simulink model "Simulacoes_lineares_naolineares"  (R2023b)
settings: Solver=ode14x  StartTime=0.0  StopTime=100  FixedStep=0.001  MaxStep=0.001  RelTol=1e-3  AbsTol=1e-3
values from neighbouring files (symbols this model uses):
  c = 0.002644555192158    (= 0.00264455519216)    [Funcoes_transferencia.m]
  carro = [K/((s+a)*(s+b))]/1000    [Funcoes_transferencia.m]
  Controlo_angulo = (46.092*(s+0.3686)*(s+5.276))/s    [Funcoes_transferencia.m]
  g = 9.8    [Funcoes_transferencia.m]
  J = 0.0001    [Funcoes_transferencia.m]
  Kd = -26.257    [Funcoes_transferencia.m]
  Kp = -26.257*6    (= -157.542)    [Funcoes_transferencia.m]
  l = 0.38    [Funcoes_transferencia.m]
  m = 0.099    [Funcoes_transferencia.m]
  s = tf('s')    [Funcoes_transferencia.m]
libraries: slpidlib x4, cstblocks x3, simulink_extras x2
settings Model: Creator=henri  LastModifiedBy=alexa
settings SolverCC: AutoScaleAbsTol=off  AlgebraicLoopSolver=TrustRegion  MaxZcPerStep=1
settings DebuggingCC: UnconnectedInputMsg=warning  UnconnectedOutputMsg=warning  UnconnectedLineMsg=warning  SymbolicDimsDataTypeCodeGenerationDiagnostic=none
settings ModelReferenceCC: EnableRefExpFcnMdlSchedulingChecks=on
settings SFSimCC: CustomCodeUndefinedFunction=UseInterfaceOnly
settings RTWCC: DLArmComputeVersion=19.05
settings SimscapeCC: SimscapeLogType=all  SimscapeLogSimulationStatistics=on  SimscapeLogDataHistory=10000

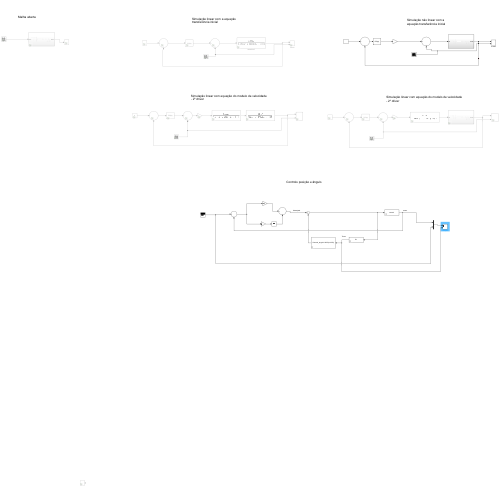
[thumbnail: Simulink's stored preview of the top-level diagram]
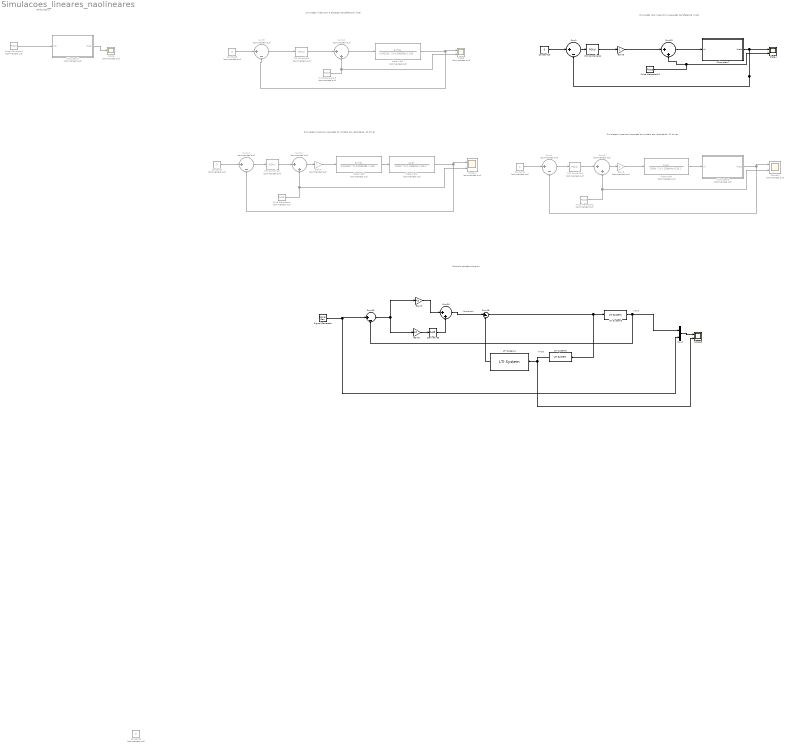
== system Simulacoes_lineares_naolineares ==
  note: Simulação linear com a equação transferência inicial
  note: Malha aberta
  note: Simulação linear com equação do modelo de velocidade - 2º driver
  note: Xdesejado
  note: Theta
  note: xcarro
  note: Controlo posição e ângulo
  note: Simulação não linear com a equação transferência inicial
  note: Simulação linear com equação do modelo de velocidade - 2º driver
  Constant{1,5..6,9} (4 alike) : Constant  Commented=on  Value=0
  Constant10 : Constant  Value=0
  Derivative3 : Derivative
  Gain4 : Gain  Commented=on
  Gain5 : Gain  Gain=Kp
  Gain6 : Gain  Gain=Kd
  Gain8 : Gain
  Gain9 : Gain  Commented=on
  LTI System3 : cstblocks/LTI System  sys=G1  IC=[]  PadeOrder=0
  LTI System4 : cstblocks/LTI System  sys=Controlo_angulo*1000/(s+1000)  IC=[]  PadeOrder=0
  LTI System5 : cstblocks/LTI System  sys=carro/s  IC=[]  PadeOrder=0
  Mux2 : Mux  Inputs=2
  PID Controller1 : slpidlib/PID Controller  Commented=on  Controller=PID  Form=Parallel  TimeDomain=Continuous-time  UseExternalTs=off  SampleTime=-1  IntegratorMethod=Forward Euler  FilterMethod=Forward Euler  ControllerParametersSource=internal  P=260.2  I=89.64  UseKiTs=off  D=46.09  N=1000  UseFilter=on  TunerSelectOption=Frequency Response Based  InitialConditionSource=internal  InitialConditionForIntegrator=0  InitialConditionForFilter=0  DifferentiatorICPrevScaledInput=0  ExternalReset=none  TrackingMode=off  Kt=1  LimitOutput=off  SatLimitsSource=internal  UpperSaturationLimit=inf  LowerSaturationLimit=-inf  LinearizeAsGain=on  AntiWindupMode=none  Kb=1  LimitIntegrator=off  UpperIntegratorSaturationLimit=inf  LowerIntegratorSaturationLimit=-inf  POutMin=[]  POutMax=[]  IOutMin=[]  IOutMax=[]  DOutMin=[]  DOutMax=[]  NOutMin=[]  NOutMax=[]  SumOutMin=[]  SumOutMax=[]  SaturationOutMin=[]  SaturationOutMax=[]  PParamMin=[]  PParamMax=[]  IParamMin=[]  IParamMax=[]  DParamMin=[]  DParamMax=[]  NParamMin=[]  NParamMax=[]  KbParamMin=[]  KbParamMax=[]  KtParamMin=[]  KtParamMax=[]  KbOutMin=[]  KbOutMax=[]  KtOutMin=[]  KtOutMax=[]  IntegratorOutMin=[]  IntegratorOutMax=[]  FilterOutMin=[]  FilterOutMax=[]  SumI1OutMin=[]  SumI1OutMax=[]  SumI2OutMin=[]  SumI2OutMax=[]  SumI3OutMin=[]  SumI3OutMax=[]  SumI4OutMin=[]  SumI4OutMax=[]  SumDOutMin=[]  SumDOutMax=[]  DifferentiatorOutMin=[]  DifferentiatorOutMax=[]  FilterDiffOutCoefMin=[]  FilterDiffOutCoefMax=[]  ReciprocalOutMin=[]  ReciprocalOutMax=[]  SumDenOutMin=[]  SumDenOutMax=[]  SumNumOutMin=[]  SumNumOutMax=[]  DivideOutMin=[]  DivideOutMax=[]  UdiffTsProdOutMin=[]  UdiffTsProdOutMax=[]  NTsProdOutMin=[]  NTsProdOutMax=[]  UintegralTsProdOutMin=[]  UintegralTsProdOutMax=[]  UngainTsProdOutMin=[]  UngainTsProdOutMax=[]  ClampingZeroOutDataTypeStr=Inherit: Inherit via back propagation  ClampingZeroOutMin=[]  ClampingZeroOutMax=[]  FilterDenConstantOutDataTypeStr=Inherit: Inherit via back propagation  FilterDenConstantOutMin=[]  FilterDenConstantOutMax=[]  PCopyOutDataTypeStr=Inherit: Inherit via back propagation  PCopyOutMin=[]  PCopyOutMax=[]  NCopyOutDataTypeStr=Inherit: Inherit via back propagation  NCopyOutMin=[]  NCopyOutMax=[]  IntegratorContinuousStateAttributes='s'  IntegratorStateMustResolveToSignalObject=off  IntegratorRTWStateStorageClass=Auto  FilterContinuousStateAttributes=''  FilterStateMustResolveToSignalObject=off  FilterRTWStateStorageClass=Auto  ParallelPVariant=InternalParameters  IdealPVariant=Disabled  IVariant=InternalParameters  DVariant=InternalParameters  IntegratorVariant=Continuous  SatVariant=Disabled  AWVariant=Passthrough  PCopyVariant=Disabled  TRVariant=Disabled  FdbkBlocksVariant=Forward  IdealPFdbkVariant=Disabled  SatFdbkVariant=Disabled  DerivativeFilterVariant=ContFilter  NVariant=InternalParameters  NCopyVariant=Disabled  FilterICVariant=InternalICsFilter  IntegratorICVariant=InternalICs  ExternalResetVariant=Disabled  TRSumVariant=Passthrough  SumFdbkVariant=Disabled  SumVariant=Sum_PID  TsampFilterVariant=InternalTs  TsampNgainVariant=Passthrough  TsampIntegralVariant=Disabled_SignalSpec  ExternalSaturationOutDataTypeStr=Inherit: Same as second input
  PID Controller11 : slpidlib/PID Controller  Controller=PID  Form=Parallel  TimeDomain=Continuous-time  UseExternalTs=off  SampleTime=-1  IntegratorMethod=Forward Euler  FilterMethod=Forward Euler  ControllerParametersSource=internal  P=1.179  I=3.284  UseKiTs=off  D=0.1053  N=1000  UseFilter=on  TunerSelectOption=Frequency Response Based  InitialConditionSource=internal  InitialConditionForIntegrator=0  InitialConditionForFilter=0  DifferentiatorICPrevScaledInput=0  ExternalReset=none  TrackingMode=off  Kt=1  LimitOutput=off  SatLimitsSource=internal  UpperSaturationLimit=inf  LowerSaturationLimit=-inf  LinearizeAsGain=on  AntiWindupMode=none  Kb=1  LimitIntegrator=off  UpperIntegratorSaturationLimit=inf  LowerIntegratorSaturationLimit=-inf  POutMin=[]  POutMax=[]  IOutMin=[]  IOutMax=[]  DOutMin=[]  DOutMax=[]  NOutMin=[]  NOutMax=[]  SumOutMin=[]  SumOutMax=[]  SaturationOutMin=[]  SaturationOutMax=[]  PParamMin=[]  PParamMax=[]  IParamMin=[]  IParamMax=[]  DParamMin=[]  DParamMax=[]  NParamMin=[]  NParamMax=[]  KbParamMin=[]  KbParamMax=[]  KtParamMin=[]  KtParamMax=[]  KbOutMin=[]  KbOutMax=[]  KtOutMin=[]  KtOutMax=[]  IntegratorOutMin=[]  IntegratorOutMax=[]  FilterOutMin=[]  FilterOutMax=[]  SumI1OutMin=[]  SumI1OutMax=[]  SumI2OutMin=[]  SumI2OutMax=[]  SumI3OutMin=[]  SumI3OutMax=[]  SumI4OutMin=[]  SumI4OutMax=[]  SumDOutMin=[]  SumDOutMax=[]  DifferentiatorOutMin=[]  DifferentiatorOutMax=[]  FilterDiffOutCoefMin=[]  FilterDiffOutCoefMax=[]  ReciprocalOutMin=[]  ReciprocalOutMax=[]  SumDenOutMin=[]  SumDenOutMax=[]  SumNumOutMin=[]  SumNumOutMax=[]  DivideOutMin=[]  DivideOutMax=[]  UdiffTsProdOutMin=[]  UdiffTsProdOutMax=[]  NTsProdOutMin=[]  NTsProdOutMax=[]  UintegralTsProdOutMin=[]  UintegralTsProdOutMax=[]  UngainTsProdOutMin=[]  UngainTsProdOutMax=[]  ClampingZeroOutDataTypeStr=Inherit: Inherit via back propagation  ClampingZeroOutMin=[]  ClampingZeroOutMax=[]  FilterDenConstantOutDataTypeStr=Inherit: Inherit via back propagation  FilterDenConstantOutMin=[]  FilterDenConstantOutMax=[]  PCopyOutDataTypeStr=Inherit: Inherit via back propagation  PCopyOutMin=[]  PCopyOutMax=[]  NCopyOutDataTypeStr=Inherit: Inherit via back propagation  NCopyOutMin=[]  NCopyOutMax=[]  IntegratorContinuousStateAttributes='s'  IntegratorStateMustResolveToSignalObject=off  IntegratorRTWStateStorageClass=Auto  FilterContinuousStateAttributes=''  FilterStateMustResolveToSignalObject=off  FilterRTWStateStorageClass=Auto  ParallelPVariant=InternalParameters  IdealPVariant=Disabled  IVariant=InternalParameters  DVariant=InternalParameters  IntegratorVariant=Continuous  SatVariant=Disabled  AWVariant=Passthrough  PCopyVariant=Disabled  TRVariant=Disabled  FdbkBlocksVariant=Forward  IdealPFdbkVariant=Disabled  SatFdbkVariant=Disabled  DerivativeFilterVariant=ContFilter  NVariant=InternalParameters  NCopyVariant=Disabled  FilterICVariant=InternalICsFilter  IntegratorICVariant=InternalICs  ExternalResetVariant=Disabled  TRSumVariant=Passthrough  SumFdbkVariant=Disabled  SumVariant=Sum_PID  TsampFilterVariant=InternalTs  TsampNgainVariant=Passthrough  TsampIntegralVariant=Disabled_SignalSpec  ExternalSaturationOutDataTypeStr=Inherit: Same as second input
  PID Controller6 : slpidlib/PID Controller  Commented=on  Controller=PID  Form=Parallel  TimeDomain=Continuous-time  UseExternalTs=off  SampleTime=-1  IntegratorMethod=Forward Euler  FilterMethod=Forward Euler  ControllerParametersSource=internal  P=1.179  I=3.284  UseKiTs=off  D=0.1053  N=1000  UseFilter=on  TunerSelectOption=Frequency Response Based  InitialConditionSource=internal  InitialConditionForIntegrator=0  InitialConditionForFilter=0  DifferentiatorICPrevScaledInput=0  ExternalReset=none  TrackingMode=off  Kt=1  LimitOutput=off  SatLimitsSource=internal  UpperSaturationLimit=inf  LowerSaturationLimit=-inf  LinearizeAsGain=on  AntiWindupMode=none  Kb=1  LimitIntegrator=off  UpperIntegratorSaturationLimit=inf  LowerIntegratorSaturationLimit=-inf  POutMin=[]  POutMax=[]  IOutMin=[]  IOutMax=[]  DOutMin=[]  DOutMax=[]  NOutMin=[]  NOutMax=[]  SumOutMin=[]  SumOutMax=[]  SaturationOutMin=[]  SaturationOutMax=[]  PParamMin=[]  PParamMax=[]  IParamMin=[]  IParamMax=[]  DParamMin=[]  DParamMax=[]  NParamMin=[]  NParamMax=[]  KbParamMin=[]  KbParamMax=[]  KtParamMin=[]  KtParamMax=[]  KbOutMin=[]  KbOutMax=[]  KtOutMin=[]  KtOutMax=[]  IntegratorOutMin=[]  IntegratorOutMax=[]  FilterOutMin=[]  FilterOutMax=[]  SumI1OutMin=[]  SumI1OutMax=[]  SumI2OutMin=[]  SumI2OutMax=[]  SumI3OutMin=[]  SumI3OutMax=[]  SumI4OutMin=[]  SumI4OutMax=[]  SumDOutMin=[]  SumDOutMax=[]  DifferentiatorOutMin=[]  DifferentiatorOutMax=[]  FilterDiffOutCoefMin=[]  FilterDiffOutCoefMax=[]  ReciprocalOutMin=[]  ReciprocalOutMax=[]  SumDenOutMin=[]  SumDenOutMax=[]  SumNumOutMin=[]  SumNumOutMax=[]  DivideOutMin=[]  DivideOutMax=[]  UdiffTsProdOutMin=[]  UdiffTsProdOutMax=[]  NTsProdOutMin=[]  NTsProdOutMax=[]  UintegralTsProdOutMin=[]  UintegralTsProdOutMax=[]  UngainTsProdOutMin=[]  UngainTsProdOutMax=[]  ClampingZeroOutDataTypeStr=Inherit: Inherit via back propagation  ClampingZeroOutMin=[]  ClampingZeroOutMax=[]  FilterDenConstantOutDataTypeStr=Inherit: Inherit via back propagation  FilterDenConstantOutMin=[]  FilterDenConstantOutMax=[]  PCopyOutDataTypeStr=Inherit: Inherit via back propagation  PCopyOutMin=[]  PCopyOutMax=[]  NCopyOutDataTypeStr=Inherit: Inherit via back propagation  NCopyOutMin=[]  NCopyOutMax=[]  IntegratorContinuousStateAttributes='s'  IntegratorStateMustResolveToSignalObject=off  IntegratorRTWStateStorageClass=Auto  FilterContinuousStateAttributes=''  FilterStateMustResolveToSignalObject=off  FilterRTWStateStorageClass=Auto  ParallelPVariant=InternalParameters  IdealPVariant=Disabled  IVariant=InternalParameters  DVariant=InternalParameters  IntegratorVariant=Continuous  SatVariant=Disabled  AWVariant=Passthrough  PCopyVariant=Disabled  TRVariant=Disabled  FdbkBlocksVariant=Forward  IdealPFdbkVariant=Disabled  SatFdbkVariant=Disabled  DerivativeFilterVariant=ContFilter  NVariant=InternalParameters  NCopyVariant=Disabled  FilterICVariant=InternalICsFilter  IntegratorICVariant=InternalICs  ExternalResetVariant=Disabled  TRSumVariant=Passthrough  SumFdbkVariant=Disabled  SumVariant=Sum_PID  TsampFilterVariant=InternalTs  TsampNgainVariant=Passthrough  TsampIntegralVariant=Disabled_SignalSpec  ExternalSaturationOutDataTypeStr=Inherit: Same as second input
  PID Controller7 : slpidlib/PID Controller  Commented=on  Controller=PID  Form=Parallel  TimeDomain=Continuous-time  UseExternalTs=off  SampleTime=-1  IntegratorMethod=Forward Euler  FilterMethod=Forward Euler  ControllerParametersSource=internal  P=260.2  I=89.64  UseKiTs=off  D=46.09  N=1000  UseFilter=on  TunerSelectOption=Frequency Response Based  InitialConditionSource=internal  InitialConditionForIntegrator=0  InitialConditionForFilter=0  DifferentiatorICPrevScaledInput=0  ExternalReset=none  TrackingMode=off  Kt=1  LimitOutput=off  SatLimitsSource=internal  UpperSaturationLimit=inf  LowerSaturationLimit=-inf  LinearizeAsGain=on  AntiWindupMode=none  Kb=1  LimitIntegrator=off  UpperIntegratorSaturationLimit=inf  LowerIntegratorSaturationLimit=-inf  POutMin=[]  POutMax=[]  IOutMin=[]  IOutMax=[]  DOutMin=[]  DOutMax=[]  NOutMin=[]  NOutMax=[]  SumOutMin=[]  SumOutMax=[]  SaturationOutMin=[]  SaturationOutMax=[]  PParamMin=[]  PParamMax=[]  IParamMin=[]  IParamMax=[]  DParamMin=[]  DParamMax=[]  NParamMin=[]  NParamMax=[]  KbParamMin=[]  KbParamMax=[]  KtParamMin=[]  KtParamMax=[]  KbOutMin=[]  KbOutMax=[]  KtOutMin=[]  KtOutMax=[]  IntegratorOutMin=[]  IntegratorOutMax=[]  FilterOutMin=[]  FilterOutMax=[]  SumI1OutMin=[]  SumI1OutMax=[]  SumI2OutMin=[]  SumI2OutMax=[]  SumI3OutMin=[]  SumI3OutMax=[]  SumI4OutMin=[]  SumI4OutMax=[]  SumDOutMin=[]  SumDOutMax=[]  DifferentiatorOutMin=[]  DifferentiatorOutMax=[]  FilterDiffOutCoefMin=[]  FilterDiffOutCoefMax=[]  ReciprocalOutMin=[]  ReciprocalOutMax=[]  SumDenOutMin=[]  SumDenOutMax=[]  SumNumOutMin=[]  SumNumOutMax=[]  DivideOutMin=[]  DivideOutMax=[]  UdiffTsProdOutMin=[]  UdiffTsProdOutMax=[]  NTsProdOutMin=[]  NTsProdOutMax=[]  UintegralTsProdOutMin=[]  UintegralTsProdOutMax=[]  UngainTsProdOutMin=[]  UngainTsProdOutMax=[]  ClampingZeroOutDataTypeStr=Inherit: Inherit via back propagation  ClampingZeroOutMin=[]  ClampingZeroOutMax=[]  FilterDenConstantOutDataTypeStr=Inherit: Inherit via back propagation  FilterDenConstantOutMin=[]  FilterDenConstantOutMax=[]  PCopyOutDataTypeStr=Inherit: Inherit via back propagation  PCopyOutMin=[]  PCopyOutMax=[]  NCopyOutDataTypeStr=Inherit: Inherit via back propagation  NCopyOutMin=[]  NCopyOutMax=[]  IntegratorContinuousStateAttributes='s'  IntegratorStateMustResolveToSignalObject=off  IntegratorRTWStateStorageClass=Auto  FilterContinuousStateAttributes=''  FilterStateMustResolveToSignalObject=off  FilterRTWStateStorageClass=Auto  ParallelPVariant=InternalParameters  IdealPVariant=Disabled  IVariant=InternalParameters  DVariant=InternalParameters  IntegratorVariant=Continuous  SatVariant=Disabled  AWVariant=Passthrough  PCopyVariant=Disabled  TRVariant=Disabled  FdbkBlocksVariant=Forward  IdealPFdbkVariant=Disabled  SatFdbkVariant=Disabled  DerivativeFilterVariant=ContFilter  NVariant=InternalParameters  NCopyVariant=Disabled  FilterICVariant=InternalICsFilter  IntegratorICVariant=InternalICs  ExternalResetVariant=Disabled  TRSumVariant=Passthrough  SumFdbkVariant=Disabled  SumVariant=Sum_PID  TsampFilterVariant=InternalTs  TsampNgainVariant=Passthrough  TsampIntegralVariant=Disabled_SignalSpec  ExternalSaturationOutDataTypeStr=Inherit: Same as second input
  Pulse Generator1 : DiscretePulseGenerator  Commented=on  PulseType=Time based  Amplitude=0.1  Period=10
  Pulse Generator11 : DiscretePulseGenerator  PulseType=Time based  Amplitude=0.1  Period=10
  Pulse Generator2 : DiscretePulseGenerator  Commented=on  PulseType=Time based  Amplitude=0.1  Period=20
  Pulse Generator5 : DiscretePulseGenerator  Commented=on  PulseType=Time based  Amplitude=0.1
  Pulse Generator6 : DiscretePulseGenerator  Commented=on  PulseType=Time based  Amplitude=0.1  Period=10
  Scope : Scope  Commented=on
  Scope1 : Scope  Commented=on  NumInputPorts=2
  Scope10 : Scope  Commented=on  NumInputPorts=2
  Scope8 : Scope  NumInputPorts=2
  Signal Generator : SignalGenerator  WaveForm=square  Amplitude=0.01  Frequency=0.04
  Subsystem1 : Subsystem  Commented=on
  Subsystem7 : Subsystem
  Subsystem8 : Subsystem  Commented=on
  Sum1 : Sum  Inputs=|+-
  Sum10 : Sum  Commented=on  Inputs=|++
  Sum11 : Sum  Commented=on  Inputs=|+-
  Sum12 : Sum  Commented=on  Inputs=|++
  Sum18 : Sum  Inputs=|+-
  Sum19 : Sum  Inputs=|+-
  Sum2 : Sum  Commented=on  Inputs=|+-
  Sum20 : Sum  Inputs=|++
  Sum23 : Sum  Inputs=|++
  Sum3 : Sum  Commented=on  Inputs=|++
  Sum9 : Sum  Commented=on  Inputs=|+-
  theta/Vref1 : TransferFcn  Commented=on  Numerator=[6.772 0]  Denominator=[0.04523 0.008308 -1.158]
  theta/Vref2 : TransferFcn  Commented=on  Numerator=[0 11.67]  Denominator=[1000 1.138e04 126.2]
  theta/Vref3 : TransferFcn  Commented=on  Numerator=[6.772 0]  Denominator=[0.04523 0.008308 -1.158]
  theta/Vref4 : TransferFcn  Commented=on  Numerator=[0 11.67]  Denominator=[1000 1.138e04 126.2]
  theta4 : Scope  NumInputPorts=2
  theta5 : Scope  Commented=on  NumInputPorts=2
  wires:
  Subsystem1/1(theta) -> Scope/1
  Pulse Generator5/1 -> theta5/2, Sum10/2
  theta/Vref1/1 -> Sum9/2, theta5/1
  Constant5/1 -> Sum9/1
  Sum9/1 -> PID Controller6/1
  PID Controller6/1 -> Sum10/1
  Sum10/1 -> theta/Vref1/1
  Pulse Generator2/1 -> Subsystem1/1(ddx)
  Gain4/1 -> theta/Vref3/1
  Sum11/1 -> PID Controller7/1
  Constant6/1 -> Sum11/1
  PID Controller7/1 -> Sum12/1
  Sum12/1 -> Gain4/1
  Pulse Generator6/1 -> Scope1/2, Sum12/2
  theta/Vref2/1 -> Sum11/2, Scope1/1
  Signal Generator/1 -> Mux2/2, Sum19/1
  Sum20/1 -> Sum18/1
  LTI System5/1 -> Mux2/1, Sum19/2
  Sum18/1 -> LTI System3/1, LTI System5/1
  Gain5/1 -> Sum20/1
  LTI System4/1 -> Sum18/2
  Gain6/1 -> Derivative3/1
  Sum19/1 -> Gain5/1, Gain6/1
  Mux2/1 -> Scope8/1
  Derivative3/1 -> Sum20/2
  LTI System3/1 -> Scope8/2, LTI System4/1
  Subsystem7/1(theta) -> Sum1/2, theta4/1
  Sum23/1 -> Subsystem7/1(dx)
  Constant10/1 -> Sum1/1
  Gain8/1 -> Sum23/1
  Sum1/1 -> PID Controller11/1
  Pulse Generator11/1 -> theta4/2, Sum23/2
  PID Controller11/1 -> Gain8/1
  theta/Vref3/1 -> theta/Vref2/1
  theta/Vref4/1 -> Subsystem8/1(dx)
  Gain9/1 -> theta/Vref4/1
  Sum3/1 -> Gain9/1
  Constant1/1 -> Sum2/1
  Sum2/1 -> PID Controller1/1
  Pulse Generator1/1 -> Scope10/2, Sum3/2
  PID Controller1/1 -> Sum3/1
  Subsystem8/1(theta) -> Sum2/2, Scope10/1

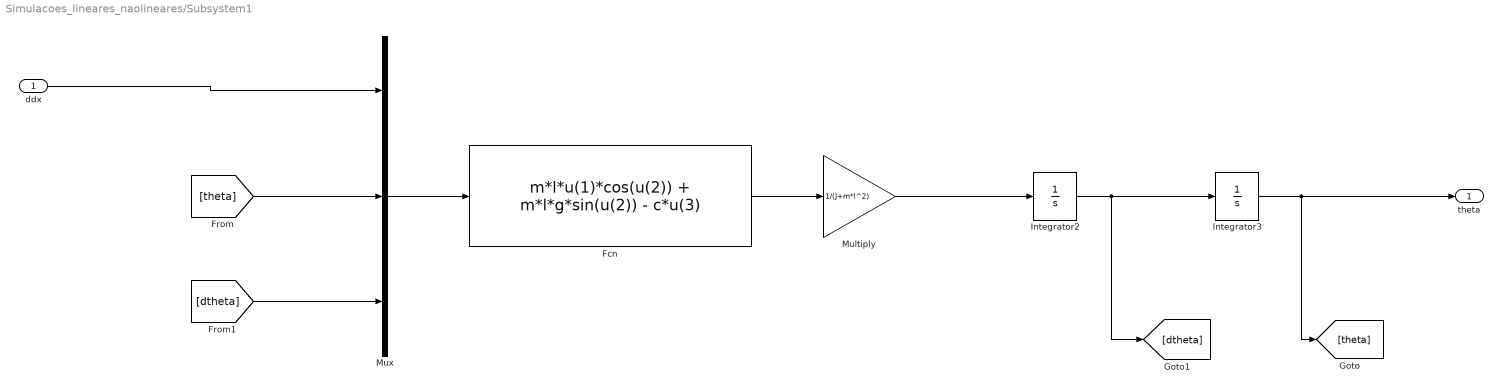
== system Simulacoes_lineares_naolineares/Subsystem1 ==
  ddx : Inport
  Fcn : Fcn  Expr=m*l*u(1)*cos(u(2)) + m*l*g*sin(u(2)) - c*u(3)
  Integrator2 : Integrator
  Integrator3 : Integrator
  Multiply : Gain  Gain=1/(J+m*l^2)
  Mux : Mux  Inputs=3
  theta : Outport
  wires:
  Fcn/1 -> Multiply/1
  [theta] -> Mux/2
  Integrator2/1 -> Integrator3/1, [dtheta]
  Mux/1 -> Fcn/1
  Integrator3/1 -> theta/1, [theta]
  Multiply/1 -> Integrator2/1
  [dtheta] -> Mux/3
  ddx/1 -> Mux/1

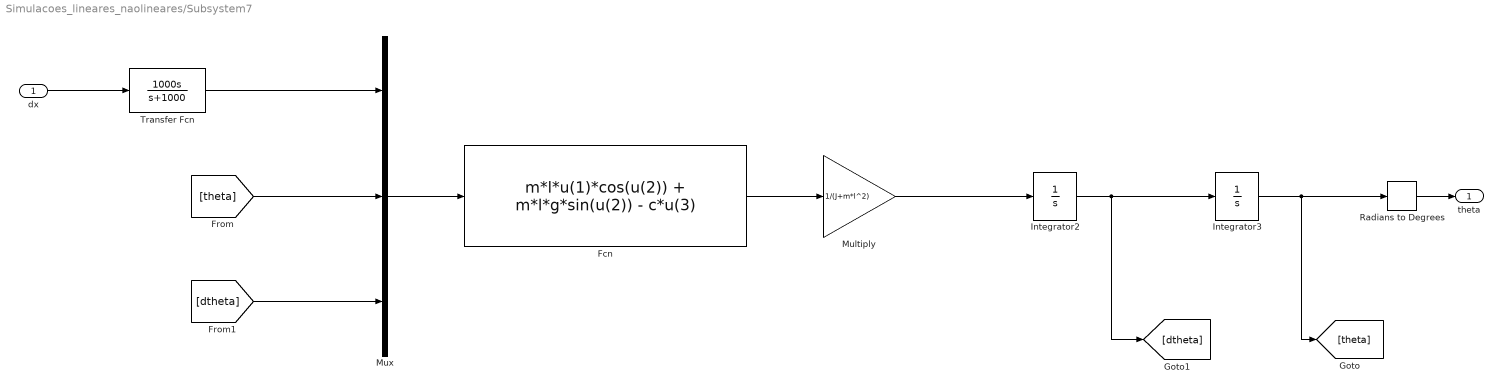
== system Simulacoes_lineares_naolineares/Subsystem7 ==
  dx : Inport
  Fcn : Fcn  Expr=m*l*u(1)*cos(u(2)) + m*l*g*sin(u(2)) - c*u(3)
  Integrator2 : Integrator
  Integrator3 : Integrator
  Multiply : Gain  Gain=1/(J+m*l^2)
  Mux : Mux  Inputs=3
  Radians to Degrees : simulink_extras/Transformations/Radians to Degrees
  Transfer Fcn : TransferFcn  Numerator=[1000 0]  Denominator=[1 1000]
  theta : Outport
  wires:
  Fcn/1 -> Multiply/1
  [theta] -> Mux/2
  Integrator2/1 -> Integrator3/1, [dtheta]
  Mux/1 -> Fcn/1
  Integrator3/1 -> Radians to Degrees/1, [theta]
  Multiply/1 -> Integrator2/1
  [dtheta] -> Mux/3
  dx/1 -> Transfer Fcn/1
  Transfer Fcn/1 -> Mux/1
  Radians to Degrees/1 -> theta/1

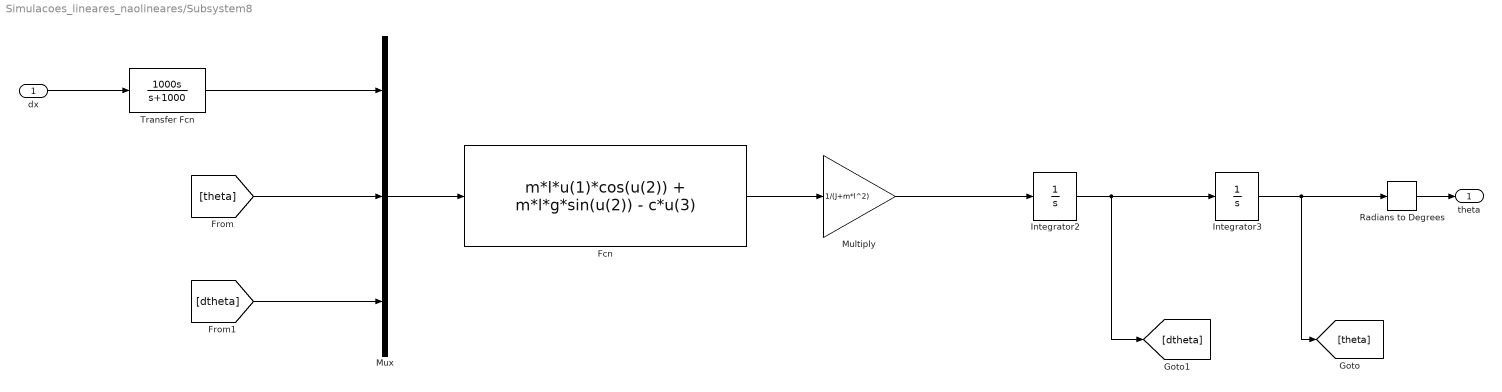
== system Simulacoes_lineares_naolineares/Subsystem8 ==
  dx : Inport
  Fcn : Fcn  Expr=m*l*u(1)*cos(u(2)) + m*l*g*sin(u(2)) - c*u(3)
  Integrator2 : Integrator
  Integrator3 : Integrator
  Multiply : Gain  Gain=1/(J+m*l^2)
  Mux : Mux  Inputs=3
  Radians to Degrees : simulink_extras/Transformations/Radians to Degrees
  Transfer Fcn : TransferFcn  Numerator=[1000 0]  Denominator=[1 1000]
  theta : Outport
  wires:
  Fcn/1 -> Multiply/1
  [theta] -> Mux/2
  Integrator2/1 -> Integrator3/1, [dtheta]
  Mux/1 -> Fcn/1
  Integrator3/1 -> Radians to Degrees/1, [theta]
  Multiply/1 -> Integrator2/1
  [dtheta] -> Mux/3
  dx/1 -> Transfer Fcn/1
  Transfer Fcn/1 -> Mux/1
  Radians to Degrees/1 -> theta/1
